simulink model "Controller_Sim"  (R2016a)
settings: Solver=ode1  SolverMode=MultiTasking  StartTime=0.0  StopTime=10  FixedStep=0.0005  RelTol=1e-3
StopFcn:
  | structifySimData
  | ConstructLog_Sim
values from neighbouring files (symbols this model uses):
  xinit = [q; dq]    [run.m]
undefined symbols (not defined in the file or in its folder): DiscIntNeverNeededParam, EnableStictionModel, FootPoints, gd, get, GroundModel, leg_length, pL1, pL2, pR1, pR2, spring_k, spring_zeta, torso_com_offset, Ts, xLine, yLine, Z
libraries: Friction_Compensator_Lib x2, robotlib x2, ControllerLibrary x1
settings Model: ParamWorkspaceSource=ReferencedWorkspace  TunableVars=AllowDoubleSupport,Alpha0Frottement,Alpha2Frottement,BoomParams,ControlParams,ControlState,ControllerModeInit,EnablePerturb,EnableTransition,EnergyControlGain,EnergyControlPhi0,GaitLibrary,HipPushMag,KASaturationEarly,KASaturationMax,KASaturationS1,KASaturationS2,KASpringOffsets,KContact,KZeroYaw,K_sha,K_sla,Ksqrt,KsqrtVert,LambdaContact,LegHipTorqueLimit,MinDeltaThetaTransition,ProjectTo2D,RunMode,SWAP_DELAY,StanceLegInit,TMaxUpdate,TPosing,TorsoBackAngle,TorsoBackOnStep,TransitionOutputParams,UseKASaturation,UsePosingControl,VBLAOptions,WalkingOutputParams,balanceParams,enable_dx_tgt,enable_dy_tgt,enable_sideStep,enable_yawControl,epsilon,ff_params,foot_adjust_params,foot_geometry,foot_points,ground_coefficient_of_friction,ground_height_data,h_alpha_nom,h_alpha_transition,hd_posing,hold_ctrl,isTest_constantHips,isTest_doubleSupport,isTest_hipTracking,isTest_holdInAir,isTest_stopAndGo,k_precomp,kd,kd_2dof,kd_ctrl,kd_hip,kd_pitch,kd_roll,kd_sha,kd_sla,kd_st_leg,kd_stanceHip,kd_stanceKnee,kd_stanceLeg,kd_sw_leg,kd_swingHip,kd_swingKnee,kd_swingLeg,kd_torso,ki_sha,ki_sla,kp,kp_2dof,kp_ctrl,kp_hip,kp_pitch,kp_roll,kp_sha,kp_sla,kp_st_leg,kp_stanceHip,kp_stanceKnee,kp_stanceLeg,kp_sw_leg,kp_swingHip,kp_swingKnee,kp_swingLeg,kp_torso,kp_yaw,lat_bias,lateralParams,optimal_sat_weights,pBInitial,ps3Axes,ps3Buttons,ps3Pov,regulate_velocity_ctrl,s_hold_ctrl,springDeflectionImpactThreshold,spring_k,spring_zeta,stepTime,step_params,swap_params,swingHipAdjustmentGain,swingLegAdjustmentGain,tStepInitial,theta_limits_nom,theta_limits_transition,thres_hi,thres_lo,torso_control_ctrl,transitionParams,uHipGravity,u_ff,use2DOFHipControl,useConstantDecoupling,useOptimalSaturation,use_state_estimator,viscous_friction_yaw_constant,w_torso_lat,xinit  TunableVarsStorageClass=Auto,Auto,Auto,Auto,Auto,Auto,Auto,Auto,Auto,Auto,Auto,Auto,Auto,Auto,Auto,Auto,Auto,Auto,Auto,Auto,Auto,Auto,Auto,Auto,Auto,Auto,Auto,Auto,Auto,Auto,Auto,Auto,Auto,Auto,Auto,Auto,Auto,Auto,Auto,Auto,Auto,Auto,Auto,Auto,Auto,Auto,Auto,Auto,Auto,Auto,Auto,Auto,Auto,Auto,Auto,Auto,Auto,Auto,Auto,Auto,Auto,Auto,Auto,Auto,Auto,Auto,Auto,Auto,Auto,Auto,Auto,Auto,Auto,Auto,Auto,Auto,Auto,Auto,Auto,Auto,Auto,Auto,Auto,Auto,Auto,Auto,Auto,Auto,Auto,Auto,Auto,Auto,Auto,Auto,Auto,Auto,Auto,Auto,Auto,Auto,Auto,Auto,Auto,Auto,Auto,Auto,Auto,Auto,Auto,Auto,Auto,Auto,Auto,Auto,Auto,Auto,Auto,Auto,Auto,Auto,Auto,Auto,Auto,Auto,Auto,Auto,Auto,Auto,Auto,Auto,Auto,Auto  TunableVarsTypeQualifier=,,,,,,,,,,,,,,,,,,,,,,,,,,,,,,,,,,,,,,,,,,,,,,,,,,,,,,,,,,,,,,,,,,,,,,,,,,,,,,,,,,,,,,,,,,,,,,,,,,,,,,,,,,,,,,,,,,,,,,,,,,,,,,,,,,,  Creator=kevinsg  LastModifiedBy=gyk
settings SolverCC: AlgebraicLoopSolver=LineSearch
settings DataIOCC: SaveFormat=Array  SaveState=on  SignalLogging=off  DSMLogging=off  TimeSaveName=t_out
settings OptimizationCC: BlockReduction=off  BooleanDataType=off
settings DebuggingCC: SaveWithParameterizedLinksMsg=none  SignalResolutionControl=TryResolveAllWithWarning  AllowSymbolicDim=off
settings HardwareCC: ProdBitPerPointer=32  ProdLargestAtomicFloat=None  ProdIntDivRoundTo=Undefined  ProdEndianess=Unspecified  ProdWordSize=32  ProdHWDeviceType=32-bit Generic  TargetBitPerPointer=64  TargetLongLongMode=on  TargetIntDivRoundTo=Zero  TargetEndianess=LittleEndian  TargetWordSize=64  TargetHWDeviceType=MATLAB Host  ProdEqTarget=off
settings ModelReferenceCC: PropagateSignalLabelsOutOfModel=off
settings RTWCC: BuildConfiguration=Faster Runs
settings ConfigComp: CovModelRefEnable=Off  CovSFcnEnable=off

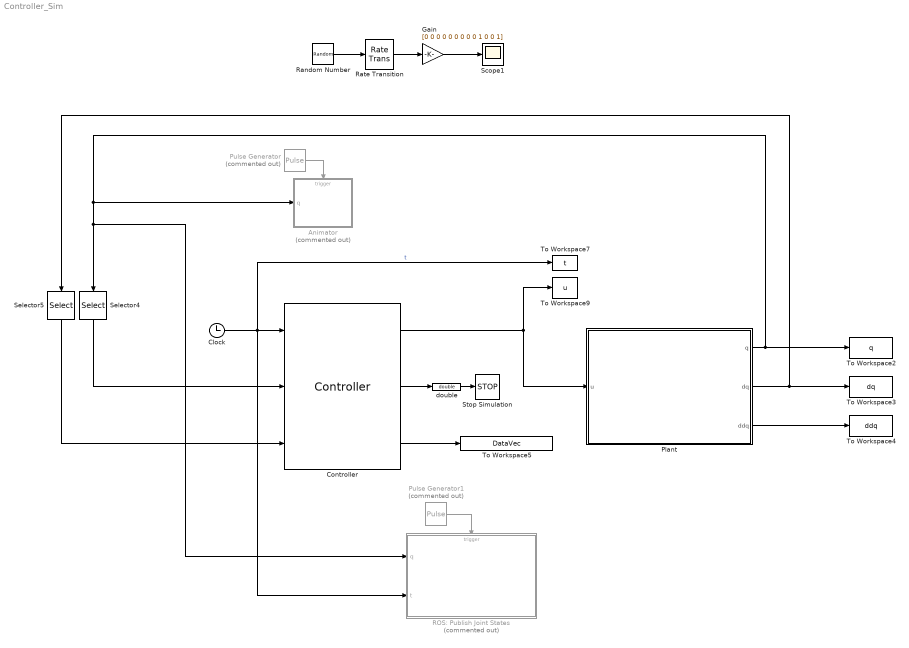
== system Controller_Sim ==
  Animator : Subsystem  Commented=on
  Clock : Clock
  Controller : ControllerLibrary/Controller
  Gain : Gain  Gain=[0 0 0 0 0 0 0 0 0 1 0 0 1]
  Plant : Subsystem
  Pulse Generator : DiscretePulseGenerator  Commented=on  PulseType=Time based  Period=.01  PulseWidth=5
  Pulse Generator1 : DiscretePulseGenerator  Commented=on  PulseType=Time based  Period=.01  PulseWidth=5
  ROS: Publish Joint States : Subsystem  Commented=on
  Random Number : RandomNumber  Variance=Ts*300  SampleTime=Ts*100
  Rate Transition : RateTransition  OutPortSampleTime=Ts
  Scope1 : Scope
  Selector4 : Selector  InputPortWidth=16  IndexOptions=Index vector (dialog)  Indices=[4,5,6,7,8,9,10,11,12,13,14,15,16]  OutputSizes=1
  Selector5 : Selector  InputPortWidth=16  IndexOptions=Index vector (dialog)  Indices=[4,5,6,7,8,9,10,11,12,13,14,15,16]  OutputSizes=1
  Stop Simulation : Stop
  To Workspace2 : ToWorkspace  VariableName=q  SampleTime=-1
  To Workspace3 : ToWorkspace  VariableName=dq  SampleTime=-1
  To Workspace4 : ToWorkspace  VariableName=ddq  SampleTime=-1
  To Workspace5 : ToWorkspace  VariableName=DataVec  SampleTime=-1
  To Workspace7 : ToWorkspace  VariableName=t  SampleTime=-1
  To Workspace9 : ToWorkspace  VariableName=u  SampleTime=-1
  double : DataTypeConversion  OutDataTypeStr=double
  wires:
  double/1 -> Stop Simulation/1
  Plant/3(ddq) -> To Workspace4/1
  Random Number/1 -> Rate Transition/1
  Rate Transition/1 -> Gain/1
  Gain/1 -> Scope1/1
  Selector4/1 -> Controller/2
  Selector5/1 -> Controller/3
  Controller/3 -> To Workspace5/1
  Controller/2 -> double/1
  Controller/1 -> To Workspace9/1, Plant/1(u)
  Pulse Generator/1 -> Animator/Trigger
  Plant/1(q) -> Selector4/1, ROS: Publish Joint States/1(q), Animator/1(q), To Workspace2/1
  Pulse Generator1/1 -> ROS: Publish Joint States/Trigger
  Plant/2(dq) -> Selector5/1, To Workspace3/1
  Clock/1 -> Controller/1, ROS: Publish Joint States/2(t), To Workspace7/1  "t"

== system Controller_Sim/Animator ==
  q : Inport
  Trigger : TriggerPort  VariantControl=Variant  PortDimensions=1
  MATLAB Function : MATLAB Function  TreatAsAtomicUnit=on
  torso_com_offset : Constant  Value=torso_com_offset
  torso_com_offset1 : Constant  Value=leg_length
  wires:
  q/1 -> MATLAB Function/1(q)
  torso_com_offset1/1 -> MATLAB Function/2(leg_length)
  torso_com_offset/1 -> MATLAB Function/3(torso_com_offset)

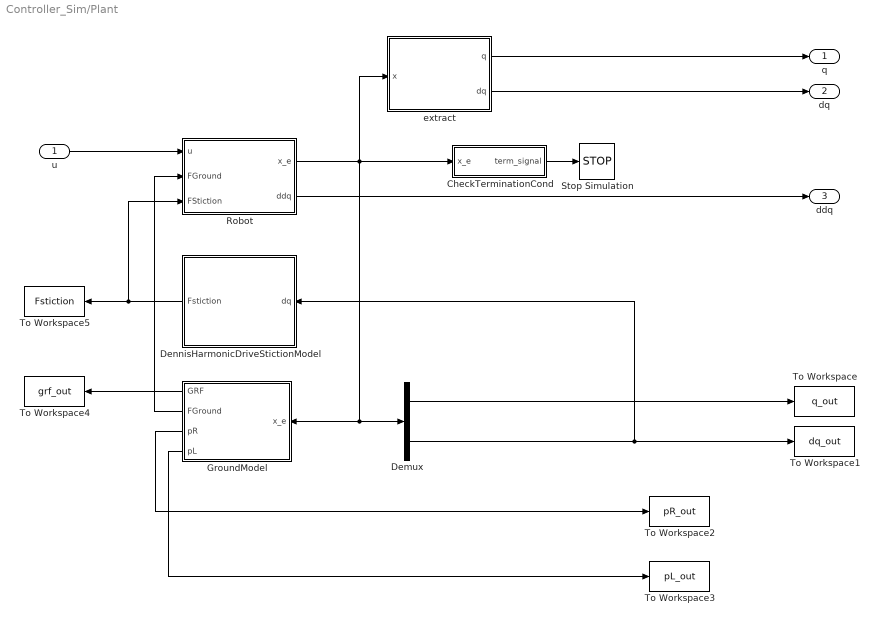
== system Controller_Sim/Plant ==
  u : Inport
  CheckTerminationCond : Subsystem
  Demux : Demux  Outputs=[16 16]
  DennisHarmonicDriveStictionModel : Subsystem
  GroundModel : Subsystem
  Robot : Subsystem
  Stop Simulation : Stop
  To Workspace : ToWorkspace  VariableName=q_out  SampleTime=-1
  To Workspace1 : ToWorkspace  VariableName=dq_out  SampleTime=-1
  To Workspace2 : ToWorkspace  VariableName=pR_out  SampleTime=-1
  To Workspace3 : ToWorkspace  VariableName=pL_out  SampleTime=-1
  To Workspace4 : ToWorkspace  VariableName=grf_out  SampleTime=-1
  To Workspace5 : ToWorkspace  VariableName=Fstiction  SampleTime=-1
  extract : MATLAB Function  TreatAsAtomicUnit=on
  q : Outport
  dq : Outport  Port=2
  ddq : Outport  Port=3
  wires:
  Robot/1(x_e) -> GroundModel/1(x_e), Demux/1, CheckTerminationCond/1(x_e), extract/1(x)
  GroundModel/2(FGround) -> Robot/2(FGround)
  Demux/2 -> DennisHarmonicDriveStictionModel/1(dq), To Workspace1/1
  Demux/1 -> To Workspace/1
  CheckTerminationCond/1(term_signal) -> Stop Simulation/1
  u/1 -> Robot/1(u)
  extract/1(q) -> q/1
  GroundModel/1(GRF) -> To Workspace4/1
  GroundModel/3(pR) -> To Workspace2/1
  GroundModel/4(pL) -> To Workspace3/1
  DennisHarmonicDriveStictionModel/1(Fstiction) -> To Workspace5/1, Robot/3(FStiction)
  extract/2(dq) -> dq/1
  Robot/2(ddq) -> ddq/1

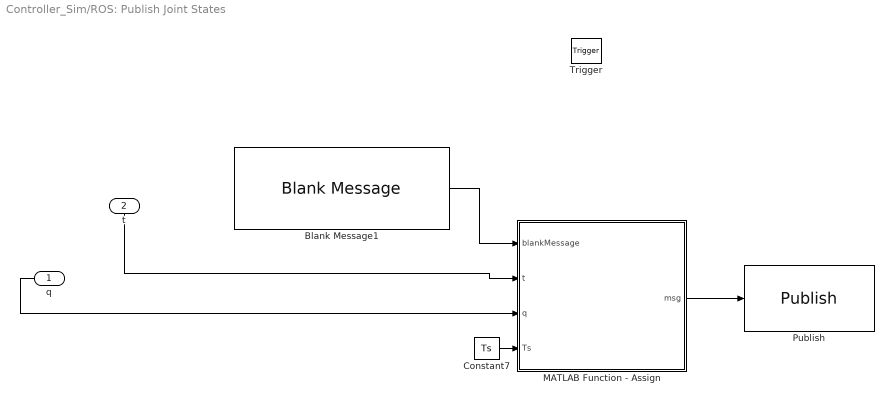
== system Controller_Sim/ROS: Publish Joint States ==
  q : Inport
  t : Inport  Port=2
  Trigger : TriggerPort  VariantControl=Variant  PortDimensions=1
  Blank Message1 : robotlib/Blank Message  SourceLibraryInfo=This block requires Robotics System Toolbox  messageType=trajectory_msgs/JointTrajectory  SampleTime=inf
  Constant7 : Constant  Value=Ts
  MATLAB Function - Assign : MATLAB Function  TreatAsAtomicUnit=on
  Publish : robotlib/Publish  SourceLibraryInfo=This block requires Robotics System Toolbox  topicSource=Specify your own  topic=/set_joint_trajectory  messageType=trajectory_msgs/JointTrajectory  messageQueueLength=1
  wires:
  MATLAB Function - Assign/1(msg) -> Publish/1
  Blank Message1/1 -> MATLAB Function - Assign/1(blankMessage)
  t/1 -> MATLAB Function - Assign/2(t)
  q/1 -> MATLAB Function - Assign/3(q)
  Constant7/1 -> MATLAB Function - Assign/4(Ts)

== system Controller_Sim/Plant/CheckTerminationCond ==
  x_e : Inport
  MATLAB Function : MATLAB Function  TreatAsAtomicUnit=on
  torso_com_offset : Constant  Value=torso_com_offset
  torso_com_offset1 : Constant  Value=leg_length
  term_signal : Outport
  wires:
  x_e/1 -> MATLAB Function/1(x_e)
  MATLAB Function/1(terminate_signal) -> term_signal/1
  torso_com_offset1/1 -> MATLAB Function/2(leg_length)
  torso_com_offset/1 -> MATLAB Function/3(torso_com_offset)

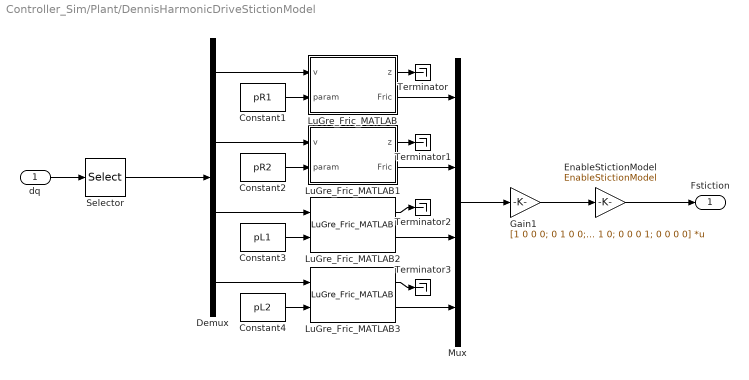
== system Controller_Sim/Plant/DennisHarmonicDriveStictionModel ==
  dq : Inport
  Constant1 : Constant  Value=pR1
  Constant2 : Constant  Value=pR2
  Constant3 : Constant  Value=pL1
  Constant4 : Constant  Value=pL2
  Demux : Demux
  EnableStictionModel : Gain  Gain=EnableStictionModel
  Gain1 : Gain  Gain=[1 0 0 0; 0 1 0 0; 0 0 0 0; 0 0 1 0; 0 0 0 1; 0 0 0 0]  Multiplication=Matrix(K*u)
  LuGre_Fric_MATLAB : Subsystem  AncestorBlock=Friction_Compensator_Lib/LuGre_Fric_MATLAB
  LuGre_Fric_MATLAB1 : Subsystem  AncestorBlock=Friction_Compensator_Lib/LuGre_Fric_MATLAB
  LuGre_Fric_MATLAB2 : Friction_Compensator_Lib/LuGre_Fric_MATLAB
  LuGre_Fric_MATLAB3 : Friction_Compensator_Lib/LuGre_Fric_MATLAB
  Mux : Mux
  Selector : Selector  InputPortWidth=16  IndexOptions=Index vector (dialog)  Indices=[11 12 14 15]  OutputSizes=1
  Terminator{,1..3} (4 alike) : Terminator
  Fstiction : Outport
  wires:
  dq/1 -> Selector/1
  Selector/1 -> Demux/1
  EnableStictionModel/1 -> Fstiction/1
  Gain1/1 -> EnableStictionModel/1
  Constant1/1 -> LuGre_Fric_MATLAB/2(param)
  Constant2/1 -> LuGre_Fric_MATLAB1/2(param)
  Constant3/1 -> LuGre_Fric_MATLAB2/2
  Constant4/1 -> LuGre_Fric_MATLAB3/2
  Demux/4 -> LuGre_Fric_MATLAB3/1
  Demux/3 -> LuGre_Fric_MATLAB2/1
  Demux/2 -> LuGre_Fric_MATLAB1/1(v)
  Demux/1 -> LuGre_Fric_MATLAB/1(v)
  LuGre_Fric_MATLAB/2(Fric) -> Mux/1
  LuGre_Fric_MATLAB1/2(Fric) -> Mux/2
  LuGre_Fric_MATLAB2/2 -> Mux/3
  LuGre_Fric_MATLAB3/2 -> Mux/4
  Mux/1 -> Gain1/1
  LuGre_Fric_MATLAB/1(z) -> Terminator/1
  LuGre_Fric_MATLAB1/1(z) -> Terminator1/1
  LuGre_Fric_MATLAB2/1 -> Terminator2/1
  LuGre_Fric_MATLAB3/1 -> Terminator3/1

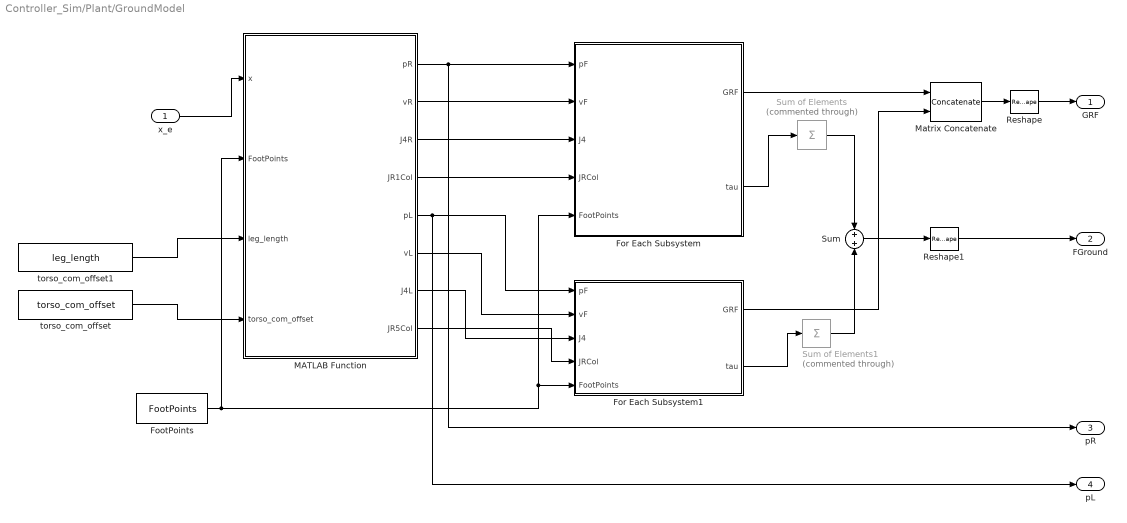
== system Controller_Sim/Plant/GroundModel ==
  x_e : Inport
  FootPoints : Constant  Value=FootPoints
  For Each Subsystem : Subsystem  TreatAsAtomicUnit=on
  For Each Subsystem1 : Subsystem  TreatAsAtomicUnit=on
  MATLAB Function : MATLAB Function  TreatAsAtomicUnit=on
  Matrix Concatenate : Concatenate  Mode=Multidimensional array
  Reshape : Reshape
  Reshape1 : Reshape
  Sum : Sum  Inputs=+|+
  Sum of Elements : Sum  Commented=through  Inputs=+  CollapseMode=Specified dimension  CollapseDim=2
  Sum of Elements1 : Sum  Commented=through  Inputs=+  CollapseMode=Specified dimension  CollapseDim=2
  torso_com_offset : Constant  Value=torso_com_offset
  torso_com_offset1 : Constant  Value=leg_length
  GRF : Outport
  FGround : Outport  Port=2
  pR : Outport  Port=3
  pL : Outport  Port=4
  wires:
  x_e/1 -> MATLAB Function/1(x)
  MATLAB Function/1(pR) -> pR/1, For Each Subsystem/1(pF)
  For Each Subsystem/1(GRF) -> Matrix Concatenate/1
  Matrix Concatenate/1 -> Reshape/1
  For Each Subsystem1/1(GRF) -> Matrix Concatenate/2
  Reshape/1 -> GRF/1
  MATLAB Function/2(vR) -> For Each Subsystem/2(vF)
  MATLAB Function/3(J4R) -> For Each Subsystem/3(J4)
  MATLAB Function/4(JR1Col) -> For Each Subsystem/4(JRCol)
  MATLAB Function/5(pL) -> For Each Subsystem1/1(pF), pL/1
  MATLAB Function/6(vL) -> For Each Subsystem1/2(vF)
  MATLAB Function/7(J4L) -> For Each Subsystem1/3(J4)
  MATLAB Function/8(JR5Col) -> For Each Subsystem1/4(JRCol)
  FootPoints/1 -> MATLAB Function/2(FootPoints), For Each Subsystem/5(FootPoints), For Each Subsystem1/5(FootPoints)
  For Each Subsystem/2(tau) -> Sum of Elements/1
  For Each Subsystem1/2(tau) -> Sum of Elements1/1
  Sum of Elements/1 -> Sum/1
  Sum of Elements1/1 -> Sum/2
  Sum/1 -> Reshape1/1
  Reshape1/1 -> FGround/1
  torso_com_offset1/1 -> MATLAB Function/3(leg_length)
  torso_com_offset/1 -> MATLAB Function/4(torso_com_offset)

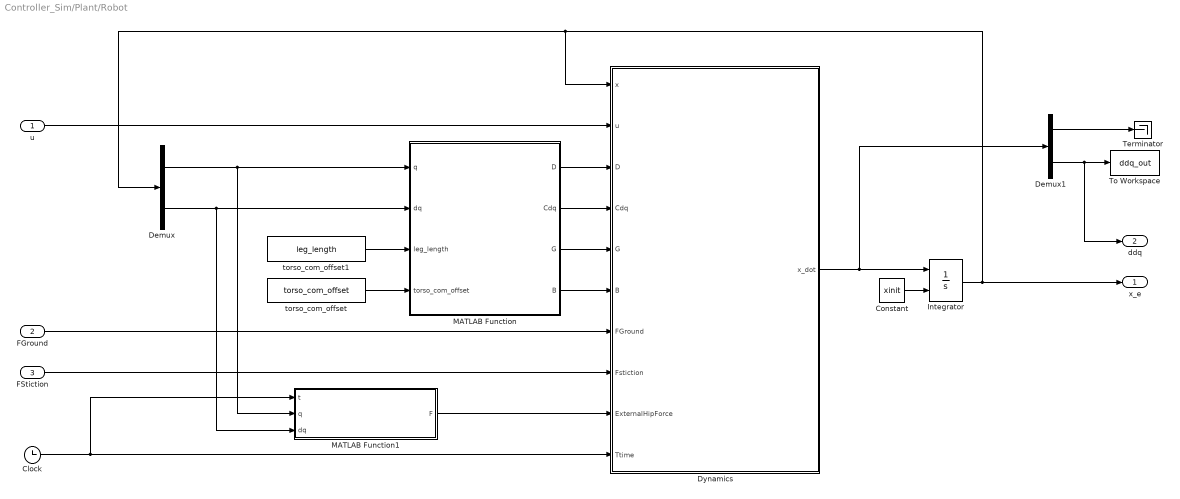
== system Controller_Sim/Plant/Robot ==
  u : Inport
  FGround : Inport  Port=2
  FStiction : Inport  Port=3
  Clock : Clock
  Constant : Constant  Value=xinit
  Demux : Demux  Outputs=[16 16]
  Demux1 : Demux  Outputs=[16 16]
  Dynamics : MATLAB Function  TreatAsAtomicUnit=on
  Integrator : Integrator  InitialConditionSource=external  InitialCondition=str2num(get(gd.edit1,'string'))
  MATLAB Function : MATLAB Function  TreatAsAtomicUnit=on
  MATLAB Function1 : MATLAB Function  TreatAsAtomicUnit=on
  Terminator : Terminator
  To Workspace : ToWorkspace  VariableName=ddq_out  SampleTime=-1
  torso_com_offset : Constant  Value=torso_com_offset
  torso_com_offset1 : Constant  Value=leg_length
  x_e : Outport
  ddq : Outport  Port=2
  wires:
  FGround/1 -> Dynamics/7(FGround)
  u/1 -> Dynamics/2(u)
  Constant/1 -> Integrator/2
  Dynamics/1(x_dot) -> Demux1/1, Integrator/1
  Clock/1 -> MATLAB Function1/1(t), Dynamics/10(Ttime)
  FStiction/1 -> Dynamics/8(Fstiction)
  MATLAB Function1/1(F) -> Dynamics/9(ExternalHipForce)
  Demux1/2 -> To Workspace/1, ddq/1
  Demux1/1 -> Terminator/1
  Demux/1 -> MATLAB Function1/2(q), MATLAB Function/1(q)
  Demux/2 -> MATLAB Function1/3(dq), MATLAB Function/2(dq)
  MATLAB Function/1(D) -> Dynamics/3(D)
  MATLAB Function/2(Cdq) -> Dynamics/4(Cdq)
  MATLAB Function/3(G) -> Dynamics/5(G)
  MATLAB Function/4(B) -> Dynamics/6(B)
  torso_com_offset/1 -> MATLAB Function/4(torso_com_offset)
  torso_com_offset1/1 -> MATLAB Function/3(leg_length)
  Integrator/1 -> Dynamics/1(x), Demux/1, x_e/1

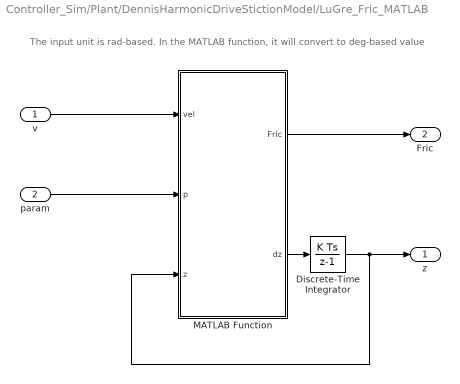
== system Controller_Sim/Plant/DennisHarmonicDriveStictionModel/LuGre_Fric_MATLAB ==
  note: The input unit is rad-based. In the MATLAB function, it will convert to deg-based value
  v : Inport
  param : Inport  Port=2
  Discrete-Time Integrator : DiscreteIntegrator  InitialConditionSetting=State (most efficient)  SampleTime=-1  ICPrevOutput=DiscIntNeverNeededParam  ICPrevScaledInput=DiscIntNeverNeededParam
  MATLAB Function : MATLAB Function  TreatAsAtomicUnit=on
  z : Outport
  Fric : Outport  Port=2
  wires:
  MATLAB Function/2(dz) -> Discrete-Time Integrator/1
  Discrete-Time Integrator/1 -> MATLAB Function/3(z), z/1
  MATLAB Function/1(Fric) -> Fric/1
  v/1 -> MATLAB Function/1(vel)
  param/1 -> MATLAB Function/2(p)

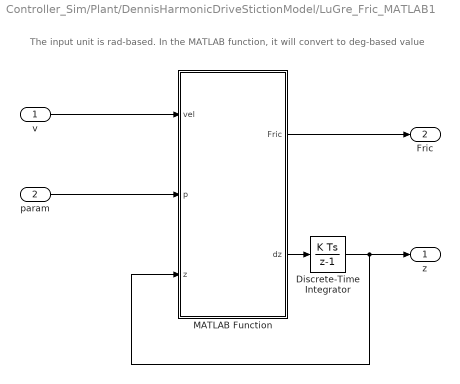
== system Controller_Sim/Plant/DennisHarmonicDriveStictionModel/LuGre_Fric_MATLAB1 ==
  note: The input unit is rad-based. In the MATLAB function, it will convert to deg-based value
  v : Inport
  param : Inport  Port=2
  Discrete-Time Integrator : DiscreteIntegrator  InitialConditionSetting=State (most efficient)  SampleTime=-1  ICPrevOutput=DiscIntNeverNeededParam  ICPrevScaledInput=DiscIntNeverNeededParam
  MATLAB Function : MATLAB Function  TreatAsAtomicUnit=on
  z : Outport
  Fric : Outport  Port=2
  wires:
  MATLAB Function/2(dz) -> Discrete-Time Integrator/1
  Discrete-Time Integrator/1 -> MATLAB Function/3(z), z/1
  MATLAB Function/1(Fric) -> Fric/1
  v/1 -> MATLAB Function/1(vel)
  param/1 -> MATLAB Function/2(p)

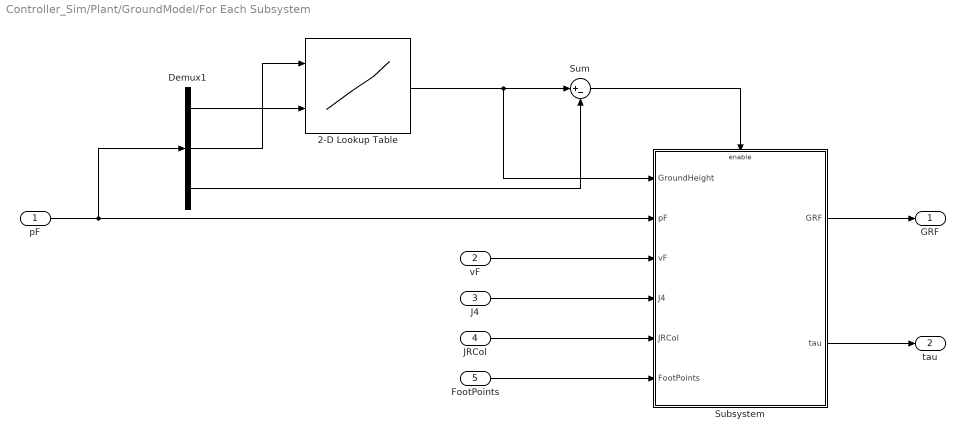
== system Controller_Sim/Plant/GroundModel/For Each Subsystem ==
  pF : Inport
  vF : Inport  Port=2
  J4 : Inport  Port=3
  JRCol : Inport  Port=4
  FootPoints : Inport  Port=5
  2-D Lookup Table : Lookup_n-D  BreakpointsForDimension1=xLine  BreakpointsForDimension2=yLine  Table=Z  InternalRulePriority=Speed  RndMeth=Simplest  InputSameDT=on
  Demux1 : Demux  Outputs=3
  Subsystem : Subsystem
  Sum : Sum  Inputs=|+-
  GRF : Outport
  tau : Outport  Port=2
  wires:
  vF/1 -> Subsystem/3(vF)
  J4/1 -> Subsystem/4(J4)
  JRCol/1 -> Subsystem/5(JRCol)
  FootPoints/1 -> Subsystem/6(FootPoints)
  Subsystem/2(tau) -> tau/1
  Sum/1 -> Subsystem/Enable
  Demux1/1 -> 2-D Lookup Table/2
  Demux1/2 -> 2-D Lookup Table/1
  pF/1 -> Subsystem/2(pF), Demux1/1
  2-D Lookup Table/1 -> Subsystem/1(GroundHeight), Sum/1
  Demux1/3 -> Sum/2
  Subsystem/1(GRF) -> GRF/1

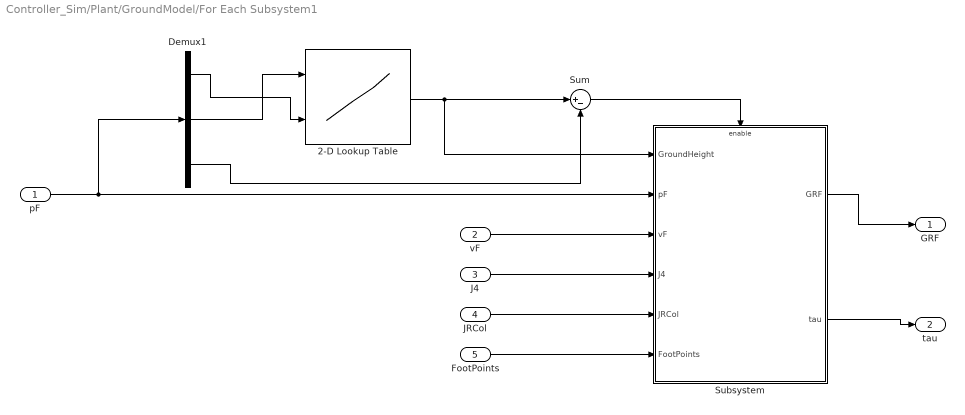
== system Controller_Sim/Plant/GroundModel/For Each Subsystem1 ==
  pF : Inport
  vF : Inport  Port=2
  J4 : Inport  Port=3
  JRCol : Inport  Port=4
  FootPoints : Inport  Port=5
  2-D Lookup Table : Lookup_n-D  BreakpointsForDimension1=xLine  BreakpointsForDimension2=yLine  Table=Z  InternalRulePriority=Speed  RndMeth=Simplest  InputSameDT=on
  Demux1 : Demux  Outputs=3
  Subsystem : Subsystem
  Sum : Sum  Inputs=|+-
  GRF : Outport
  tau : Outport  Port=2
  wires:
  Subsystem/1(GRF) -> GRF/1
  Demux1/3 -> Sum/2
  2-D Lookup Table/1 -> Sum/1, Subsystem/1(GroundHeight)
  pF/1 -> Demux1/1, Subsystem/2(pF)
  Demux1/2 -> 2-D Lookup Table/1
  Demux1/1 -> 2-D Lookup Table/2
  Sum/1 -> Subsystem/Enable
  Subsystem/2(tau) -> tau/1
  FootPoints/1 -> Subsystem/6(FootPoints)
  JRCol/1 -> Subsystem/5(JRCol)
  J4/1 -> Subsystem/4(J4)
  vF/1 -> Subsystem/3(vF)

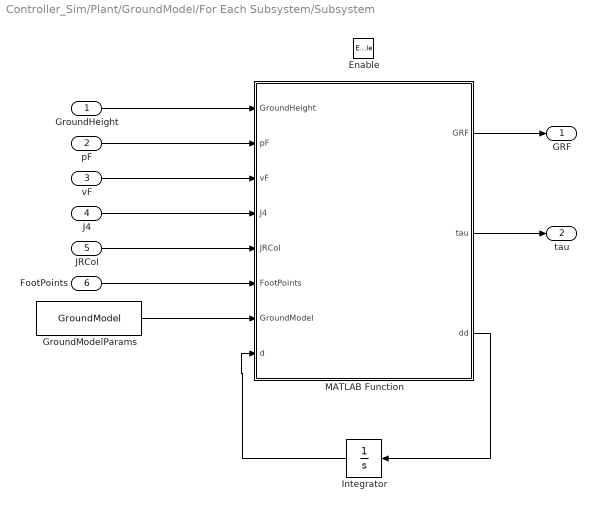
== system Controller_Sim/Plant/GroundModel/For Each Subsystem/Subsystem ==
  GroundHeight : Inport
  pF : Inport  Port=2
  vF : Inport  Port=3
  J4 : Inport  Port=4
  JRCol : Inport  Port=5
  FootPoints : Inport  Port=6
  Enable : EnablePort  StatesWhenEnabling=reset
  GroundModelParams : Constant  Value=GroundModel  OutDataTypeStr=Bus: GroundModelParamsBus
  Integrator : Integrator  InitialCondition=[0; 0]
  MATLAB Function : MATLAB Function  TreatAsAtomicUnit=on
  GRF : Outport  OutputWhenDisabled=reset  InitialOutput=[0;0;0]
  tau : Outport  Port=2  OutputWhenDisabled=reset  InitialOutput=zeros(16,1)
  wires:
  GroundModelParams/1 -> MATLAB Function/7(GroundModel)
  MATLAB Function/3(dd) -> Integrator/1
  Integrator/1 -> MATLAB Function/8(d)
  vF/1 -> MATLAB Function/3(vF)
  pF/1 -> MATLAB Function/2(pF)
  MATLAB Function/1(GRF) -> GRF/1
  MATLAB Function/2(tau) -> tau/1
  J4/1 -> MATLAB Function/4(J4)
  JRCol/1 -> MATLAB Function/5(JRCol)
  FootPoints/1 -> MATLAB Function/6(FootPoints)
  GroundHeight/1 -> MATLAB Function/1(GroundHeight)

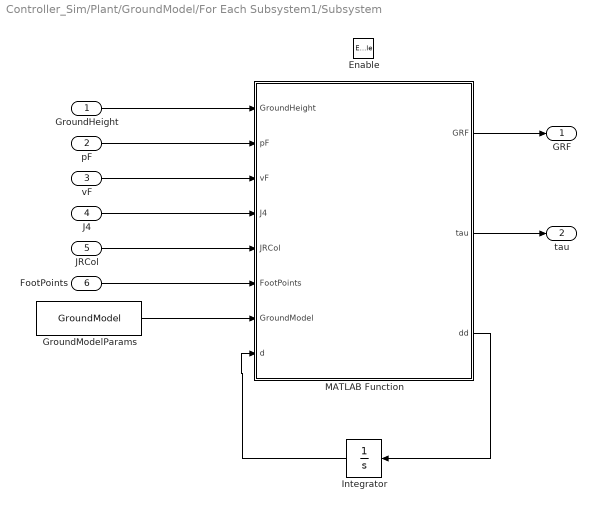
== system Controller_Sim/Plant/GroundModel/For Each Subsystem1/Subsystem ==
  GroundHeight : Inport
  pF : Inport  Port=2
  vF : Inport  Port=3
  J4 : Inport  Port=4
  JRCol : Inport  Port=5
  FootPoints : Inport  Port=6
  Enable : EnablePort  StatesWhenEnabling=reset
  GroundModelParams : Constant  Value=GroundModel  OutDataTypeStr=Bus: GroundModelParamsBus
  Integrator : Integrator  InitialCondition=[0; 0]
  MATLAB Function : MATLAB Function  TreatAsAtomicUnit=on
  GRF : Outport  OutputWhenDisabled=reset  InitialOutput=[0;0;0]
  tau : Outport  Port=2  OutputWhenDisabled=reset  InitialOutput=zeros(16,1)
  wires:
  GroundHeight/1 -> MATLAB Function/1(GroundHeight)
  FootPoints/1 -> MATLAB Function/6(FootPoints)
  JRCol/1 -> MATLAB Function/5(JRCol)
  J4/1 -> MATLAB Function/4(J4)
  MATLAB Function/2(tau) -> tau/1
  MATLAB Function/1(GRF) -> GRF/1
  pF/1 -> MATLAB Function/2(pF)
  vF/1 -> MATLAB Function/3(vF)
  Integrator/1 -> MATLAB Function/8(d)
  MATLAB Function/3(dd) -> Integrator/1
  GroundModelParams/1 -> MATLAB Function/7(GroundModel)

== matlab function Controller_Sim/Plant/GroundModel/For Each Subsystem1/Subsystem/MATLAB Function ==
  data: GroundHeight input; pF input; GRF output; tau output; vF input; J4 input; JRCol input; FootPoints input; GroundModel input; d input; dd output
function [GRF, tau, dd] = computeLuGreHertzian(GroundHeight, pF, vF, J4, JRCol, FootPoints, GroundModel, d)
    %#codegen
    
    [F, dd] = LuGreHertzian(pF(3), vF(3,:), d, vF(1:2,:), GroundModel,GroundHeight);
    GRF = F(:);
    
    J   = J4 + FootPoints(1)*JRCol(1:3,:) + FootPoints(2)*JRCol(4:6,:) + FootPoints(3)*JRCol(7:9,:);
    tau = J.'*GRF;
end

== matlab function Controller_Sim/Plant/Robot/Dynamics ==
  data: x input; u input; D input; Cdq input; G input; B input; FGround input; Fstiction input; x_dot output; spring_k parameter; spring_zeta parameter; ExternalHipForce input; Ttime input
function x_dot  = ATRIAS3D_Flight(x, u, D, Cdq, G, B, FGround, Fstiction, spring_k, spring_zeta, ExternalHipForce,Ttime)
%#codegen

q  = x(1:16);
dq = x(17:32);

% Lagrange model
%[D,Cdq,G,B,J_yaw,dJ_yaw] = ATRIAS3D_Lagrange_Hip(q,dq);

%Calculate spring and damper forces
[K_spring, K_damping] = ATRIAS3D_Spring_Constants(spring_k, spring_zeta);
FSpring = K_spring * q + K_damping * dq; 

% Calculate the H vector
H = Cdq + G + FSpring - FGround - B*(u - Fstiction)+ExternalHipForce;


ddq = -D\H;
x_dot = [dq;ddq];

%--------------------------------------------------------------------------

== matlab function Controller_Sim/Plant/GroundModel/For Each Subsystem/Subsystem/MATLAB Function ==
  data: GroundHeight input; pF input; GRF output; tau output; vF input; J4 input; JRCol input; FootPoints input; GroundModel input; d input; dd output
function [GRF, tau, dd] = computeLuGreHertzian(GroundHeight, pF, vF, J4, JRCol, FootPoints, GroundModel, d)
    %#codegen
    
    [F, dd] = LuGreHertzian(pF(3), vF(3,:), d, vF(1:2,:), GroundModel,GroundHeight);
    GRF = F(:);
    
    J   = J4 + FootPoints(1)*JRCol(1:3,:) + FootPoints(2)*JRCol(4:6,:) + FootPoints(3)*JRCol(7:9,:);
    tau = J.'*GRF;
end

== matlab function Controller_Sim/Plant/extract ==
  data: x input; q output; dq output
function [q,dq] = extract(x)
%#codegen
q = x(1:16,1);
dq = x(17:32,1);

== matlab function Controller_Sim/Plant/Robot/MATLAB Function ==
  data: q input; D output; dq input; leg_length input; Cdq output; G output; B output; torso_com_offset input
function [D, Cdq, G, B] = Compute_Lagrange_Model(q, dq, leg_length, torso_com_offset)
%#codegen

% Call functions generated from symbolic model
extra_vars = [leg_length; torso_com_offset];
D = OriginalLeg_Springs_VariableLeg_COMoffset.ATRIAS3D_D_Hip(q,extra_vars);
Cdq = OriginalLeg_Springs_VariableLeg_COMoffset.ATRIAS3D_Cdq_Hip(q,dq,extra_vars);
G = OriginalLeg_Springs_VariableLeg_COMoffset.ATRIAS3D_G_Hip(q,extra_vars);
B = OriginalLeg_Springs_VariableLeg_COMoffset.ATRIAS3D_B_Hip(q);

== matlab function Controller_Sim/Plant/Robot/MATLAB Function1 ==
  data: t input; q input; F output; dq input
function F  = ExternalForces(t, q, dq)
    F = CompliantSimulator.ExternalForces(t, q, dq);
end

== matlab function Controller_Sim/Animator/MATLAB Function ==
  data: q input; leg_length input; torso_com_offset input
function Animation(q, leg_length, torso_com_offset)
%#codegen 
persistent f p1HR p2HR p31R p42R pHR0TR p1HL p2HL p31L p42L pHR0TL torso ax
leg1Color = 'r'; 
leg2Color = 'b';
torsoColor = 'k';
groundColor = 'g';
        
% Get Positions
[pcm, p0, p0T, pHR, p1R, p2R, p3R, p4R, pHL, p1L, p2L, p3L, p4L] =  OriginalLeg_Springs_VariableLeg_COMoffset.ATRIAS3D_Positions_Hip(q,[leg_length;torso_com_offset]);

if isempty(f)
    f = figure;
    ax = axes(f);
    
    % Define stance leg
    p1HR = line(ax, [p1R(1) pHR(1)],[p1R(2) pHR(2)],[p1R(3) pHR(3)]);
    p2HR = line(ax, [p2R(1) pHR(1)],[p2R(2) pHR(2)],[p2R(3) pHR(3)]);
    p31R = line(ax, [p3R(1) p1R(1)],[p3R(2) p1R(2)],[p3R(3) p1R(3)]);
    p42R = line(ax, [p4R(1) p2R(1)],[p4R(2) p2R(2)],[p4R(3) p2R(3)]);
    pHR0TR = line(ax, [p0(1) pHR(1)],[p0(2) pHR(2)],[p0(3) pHR(3)]);
    
    set(p1HR,'LineWidth',3,'Color',leg1Color);
    set(p2HR,'LineWidth',3,'Color',leg1Color);
    set(p31R,'LineWidth',3,'Color',leg1Color);
    set(p42R,'LineWidth',3,'Color',leg1Color);
    set(pHR0TR,'LineWidth',3,'Color',torsoColor);
    
    % Define swing leg
    p1HL = line(ax, [p1L(1) pHL(1)],[p1L(2) pHL(2)],[p1L(3) pHL(3)]);
    p2HL = line(ax, [p2L(1) pHL(1)],[p2L(2) pHL(2)],[p2L(3) pHL(3)]);
    p31L = line(ax, [p3L(1) p1L(1)],[p3L(2) p1L(2)],[p3L(3) p1L(3)]);
    p42L = line(ax, [p4L(1) p2L(1)],[p4L(2) p2L(2)],[p4L(3) p2L(3)]);
    pHR0TL = line(ax, [p0(1) pHL(1)],[p0(2) pHL(2)],[p0(3) pHL(3)]);
    
    set(p1HL,'LineWidth',3,'Color',leg2Color);
    set(p2HL,'LineWidth',3,'Color',leg2Color);
    set(p31L,'LineWidth',3,'Color',leg2Color);
    set(p42L,'LineWidth',3,'Color',leg2Color);
    set(pHR0TL,'LineWidth',3,'Color',torsoColor);
    
    % Define torso
    torso = line(ax, [p0(1) p0T(1)], [p0(2) p0T(2)], [p0(3) p0T(3)]);
    set(torso,'LineWidth',3,'Color',torsoColor);

end

%figure(f);
axis(ax, [pcm(1)-1, pcm(1)+1, pcm(2)-1, pcm(2)+1, 0 2 0 1]);

set(p1HR,'XData',[p1R(1) pHR(1)],'YData',[p1R(2) pHR(2)],'ZData',[p1R(3) pHR(3)]);
set(p2HR,'XData',[p2R(1) pHR(1)],'YData',[p2R(2) pHR(2)],'ZData',[p2R(3) pHR(3)]);
set(p31R,'XData',[p3R(1) p1R(1)],'YData',[p3R(2) p1R(2)],'ZData',[p3R(3) p1R(3)]);
set(p42R,'XData',[p4R(1) p2R(1)],'YData',[p4R(2) p2R(2)],'ZData',[p4R(3) p2R(3)]);
set(pHR0TR,'XData',[p0(1) pHR(1)],'YData',[p0(2) pHR(2)],'ZData',[p0(3) pHR(3)]);

set(p1HL,'XData',[p1L(1) pHL(1)],'YData',[p1L(2) pHL(2)],'ZData',[p1L(3) pHL(3)]);
set(p2HL,'XData',[p2L(1) pHL(1)],'YData',[p2L(2) pHL(2)],'ZData',[p2L(3) pHL(3)]);
set(p31L,'XData',[p3L(1) p1L(1)],'YData',[p3L(2) p1L(2)],'ZData',[p3L(3) p1L(3)]);
set(p42L,'XData',[p4L(1) p2L(1)],'YData',[p4L(2) p2L(2)],'ZData',[p4L(3) p2L(3)]);
set(pHR0TL,'XData',[p0(1) pHL(1)],'YData',[p0(2) pHL(2)],'ZData',[p0(3) pHL(3)]);

set(torso,'XData',[p0(1) p0T(1)],'YData',[p0(2) p0T(2)],'ZData',[p0(3) p0T(3)]);

== matlab function Controller_Sim/Plant/GroundModel/MATLAB Function ==
  data: x input; pR output; vR output; J4R output; JR1Col output; pL output; vL output; J4L output; JR5Col output; FootPoints input; leg_length input; torso_com_offset input
function [pR, vR, J4R, JR1Col, pL, vL, J4L, JR5Col] = getFootHeightAndVelocity(x, FootPoints,  leg_length, torso_com_offset)
    %#codegen
    [pR, vR, J4R, JR1Col, pL, vL, J4L, JR5Col] = FootHeightAndVelocity(x, FootPoints, leg_length, torso_com_offset);
end

== matlab function Controller_Sim/Plant/CheckTerminationCond/MATLAB Function ==
  data: x_e input; terminate_signal output; leg_length input; torso_com_offset input
function terminate_signal  =  CheckTerminationConditions(x_e,leg_length,torso_com_offset)
%#codegen
%
q  = x_e(1:16);
dq = x_e(17:end);

%[pcm p0 p0T pHR p1R p2R p3R p4R pHL p1L p2L p3L p4L] = ATRIAS3D_Primary_PointsHip(q);
[pcm, p0, p0T, pHR, p1R, p2R, p3R, p4R, pHL, p1L, p2L, p3L, p4L] = OriginalLeg_Springs_VariableLeg_COMoffset.ATRIAS3D_Positions_Hip(q,[leg_length;torso_com_offset]);

p_Z = [p4L(3), p4R(3)];

%Terminate if torso top goes below 0.5m or either foot goes above 1 m
if p0T(3)<0.5 %|| max(p_Z) > 1
    terminate_signal = 1;
else    
    terminate_signal = 0;
end

== matlab function Controller_Sim/Plant/DennisHarmonicDriveStictionModel/LuGre_Fric_MATLAB/MATLAB Function ==
  data: vel input; p input; Fric output; z input; dz output
function [Fric,dz] = LuGre_Fric_MATLAB(vel,p,z)
%#codegen

% J = p(1);
alpha0 = p(2);
alpha0v2 = p(3);
alpha1 = p(4);
alpha1v2 = p(5);
alpha2 = p(6);
alpha2v2 = p(7);
alpha3 = p(8); 
alpha3v2 = p(9);
v0 = p(10);
v0v2 = p(11);
sigma0 = p(12);
sigma1 = p(13);
fConst = p(14);

x2 = vel*180/pi;
g = (alpha0+alpha1*exp(-(x2/v0).^2))*(x2>=0)+(alpha0v2+alpha1v2*exp(-(x2/v0v2).^2))*(x2<0);
dz = x2-sigma0/g*abs(x2)*z;

Fric = sigma0*z+sigma1*dz+(alpha2*x2)*(x2>=0)+(abs(alpha2v2)*x2)*(x2<0)+(alpha3*x2^2)*(x2>=0)+(-abs(alpha3v2)*x2^2)*(x2<0)+fConst;

== matlab function Controller_Sim/Plant/DennisHarmonicDriveStictionModel/LuGre_Fric_MATLAB1/MATLAB Function ==
  data: vel input; p input; Fric output; z input; dz output
function [Fric,dz] = LuGre_Fric_MATLAB(vel,p,z)
%#codegen

% J = p(1);
alpha0 = p(2);
alpha0v2 = p(3);
alpha1 = p(4);
alpha1v2 = p(5);
alpha2 = p(6);
alpha2v2 = p(7);
alpha3 = p(8); 
alpha3v2 = p(9);
v0 = p(10);
v0v2 = p(11);
sigma0 = p(12);
sigma1 = p(13);
fConst = p(14);

x2 = vel*180/pi;
g = (alpha0+alpha1*exp(-(x2/v0).^2))*(x2>=0)+(alpha0v2+alpha1v2*exp(-(x2/v0v2).^2))*(x2<0);
dz = x2-sigma0/g*abs(x2)*z;

Fric = sigma0*z+sigma1*dz+(alpha2*x2)*(x2>=0)+(abs(alpha2v2)*x2)*(x2<0)+(alpha3*x2^2)*(x2>=0)+(-abs(alpha3v2)*x2^2)*(x2<0)+fConst;

== matlab function Controller_Sim/ROS: Publish Joint States/MATLAB Function - Assign ==
  data: blankMessage input; t input; q input; msg output Bus: SL_Bus_Controller_Sim_v3_trajectory_msgs_JointTrajectory; Ts input
function msg = assign_JointTrajectory(blankMessage, t, q, Ts)
%#codegen

% To set datatype of MSG output:
%  1. Create buses for this model: robotics.ros.createSimulinkBus(gcs)
%  1. Click "Edit Data" in  Toolstrip to open "Ports and Data Manager"
%  2. Select MSG and set datatype to "Bus: SL_Bus_<modelname>_<messageType>"
% See: 
% http://www.mathworks.com/help/simulink/ug/create-structures-in-matlab-function-blocks.html

% blankMessage (nav_msgs/Odometry) consists of
%                Header: [1x1 Header]
%          ChildFrameId: variable-length array of uint8
%  ChildFrameId_SL_Info: struct with fields CurrentLength, ReceivedLength
%                  Pose: [1x1 PoseWithCovariance]
%                 Twist: [1x1 TwistWithCovariance]

% Assign the output message to be the same with input blank message
msg = blankMessage;

%% Modify the nested messages

% Assign Joint Names
strArrayToAssign = {'x', 'y', 'z', 'qz', 'qy', 'qx', 'q1R', 'q2R', 'q3R', ...
    'q1L', 'q2L', 'q3L', 'L1R_to_L4R', 'L2R_to_L3R', 'L1L_to_L4L', 'L2L_to_L3L'};
numStringsInArray = length(strArrayToAssign);
msg.JointNames_SL_Info.CurrentLength = uint32(numStringsInArray);
for idx=1:numStringsInArray
    str = strArrayToAssign{idx};
    strLength = length(str);
    msg.JointNames(idx).Data(1:strLength) = uint8(str);
    msg.JointNames(idx).Data_SL_Info.CurrentLength = uint32(strLength);
end

% Assign Frame Id
str = 'world_gazebo';
strLength = length(str);
msg.Header.FrameId_SL_Info.CurrentLength = uint32(strLength);
msg.Header.FrameId(1:strLength) = uint8(str);


% Assign Joint Positions
msg.Points_SL_Info.CurrentLength = uint32(1); 
msg.Points(1).Positions_SL_Info.CurrentLength = uint32(16);

q_vec = zeros(16,1);
q_vec(1:6) = q(1:6);
q_vec(7:12) = q([11,12,13,14,15,16]); 
q_vec(13) = (q(12) - q(11)); 
q_vec(14) = -(q(12) - q(11)); 
q_vec(15) = (q(15) - q(14)); 
q_vec(16) = -(q(15) - q(14)); 

msg.Points(1).Positions(1:16) = q_vec;
msg.Points(1).TimeFromStart.Nsec = int32(Ts/1e-9);
